simulink model "beta0"  (R2020a)
settings: Solver=VariableStepAuto  StartTime=0.0  StopTime=10.0  RelTol=1e-3
undefined symbols (not defined in the file): DiscIntNeverNeededParam
settings Model: Creator=Acer  LastModifiedBy=Acer

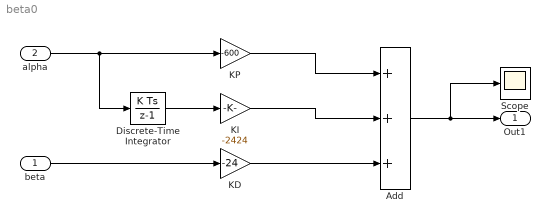
== system beta0 ==
  beta : Inport
  alpha : Inport  Port=2
  Add : Sum  Inputs=+++
  Discrete-Time Integrator : DiscreteIntegrator  SampleTime=-1  ICPrevOutput=DiscIntNeverNeededParam  ICPrevScaledInput=DiscIntNeverNeededParam
  KD : Gain  Gain=-24
  KI : Gain  Gain=-2424
  KP : Gain  Gain=-600
  Scope : Scope
  Out1 : Outport
  wires:
  beta/1 -> KD/1
  Discrete-Time Integrator/1 -> KI/1
  KD/1 -> Add/3
  KI/1 -> Add/2
  KP/1 -> Add/1
  Add/1 -> Scope/1, Out1/1
  alpha/1 -> Discrete-Time Integrator/1, KP/1
